simulink model "simulazione"  (R2021b)
settings: Solver=FixedStepAuto  StartTime=0.0  StopTime=1000  FixedStep=0.001  RelTol=1e-3
values from neighbouring files (symbols this model uses):
  b1 = 0.3    [linearizzazione.m]    (also in progetto.m)
  b2 = 0.1    [linearizzazione.m]    (also in progetto.m)
  DD = 3e-5    (= 3e-05)    [progetto.m]
  k = 1.5    [linearizzazione.m]    (also in progetto.m)
  kG = 6.67e-11    [linearizzazione.m]    (also in progetto.m)
  m = 1    [linearizzazione.m]    (also in progetto.m)
  M = 5.98e24    (= 5.98e+24)    [linearizzazione.m]    (also in progetto.m)
  u_e = 364.63    [linearizzazione.m]    (also in progetto.m)
  WW = 8e-5    (= 8e-05)    [progetto.m]
  x1_e = 3e7    (= 30000000)    [linearizzazione.m]    (also in progetto.m)
  x2_e = 0    [linearizzazione.m]    (also in progetto.m)
  x3_e = 0.000121543    [linearizzazione.m]    (also in progetto.m)
undefined symbols (not defined in the file or in its folder): NN
settings Model: Creator=lollo  LastModifiedBy=lollo

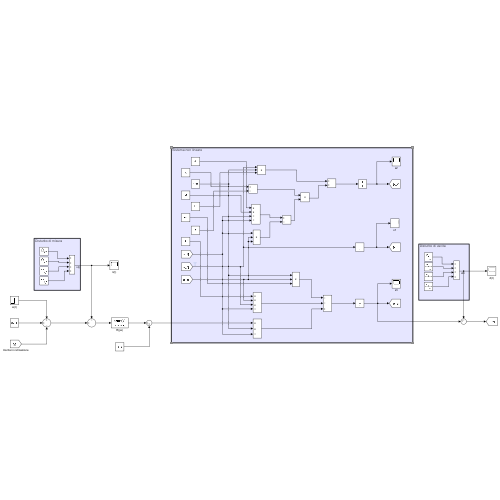
[thumbnail: Simulink's stored preview of the top-level diagram]
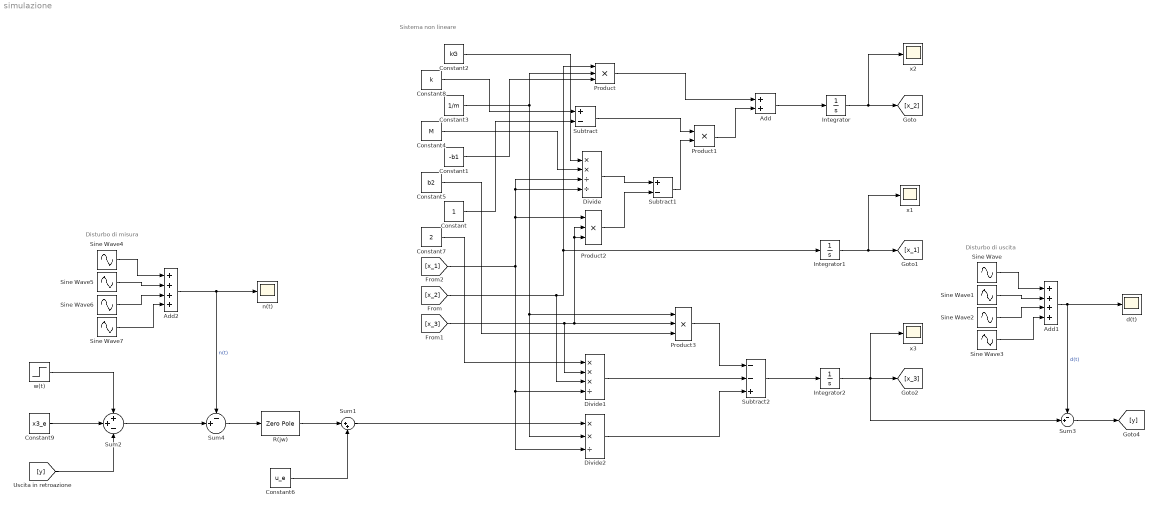
== system simulazione ==
  note: Sistema non lineare
  note: Disturbo di uscita
  note: Disturbo di misura
  Add : Sum
  Add1 : Sum  Inputs=++++
  Add2 : Sum  Inputs=++++
  Constant : Constant
  Constant1 : Constant  Value=-b1
  Constant2 : Constant  Value=kG
  Constant3 : Constant  Value=1/m
  Constant4 : Constant  Value=M
  Constant5 : Constant  Value=b2
  Constant6 : Constant  Value=u_e
  Constant7 : Constant  Value=2
  Constant8 : Constant  Value=k
  Constant9 : Constant  Value=x3_e
  Divide : Product  Inputs=**//
  Divide1 : Product  Inputs=***/
  Divide2 : Product  Inputs=**/
  Integrator : Integrator  InitialCondition=x2_e
  Integrator1 : Integrator  InitialCondition=x1_e
  Integrator2 : Integrator  InitialCondition=x3_e
  Product : Product  Inputs=3
  Product1 : Product
  Product2 : Product  Inputs=3
  Product3 : Product  Inputs=3
  R(jw) : ZeroPole  Zeros=[-0.3309]  Poles=[0 -830.2822]  Gain=2.5088e12
  Sine Wave : Sin  Amplitude=DD  Frequency=0.02*1  SampleTime=0
  Sine Wave1 : Sin  Amplitude=DD  Frequency=0.02*2  SampleTime=0
  Sine Wave2 : Sin  Amplitude=DD  Frequency=0.02*3  SampleTime=0
  Sine Wave3 : Sin  Amplitude=DD  Frequency=0.02*4  SampleTime=0
  Sine Wave4 : Sin  Amplitude=NN  Frequency=5e4*1  SampleTime=0
  Sine Wave5 : Sin  Amplitude=NN  Frequency=5e4*2  SampleTime=0
  Sine Wave6 : Sin  Amplitude=NN  Frequency=5e4*3  SampleTime=0
  Sine Wave7 : Sin  Amplitude=NN  Frequency=5e4*4  SampleTime=0
  Subtract : Sum  Inputs=+-
  Subtract1 : Sum  Inputs=+-
  Subtract2 : Sum  Inputs=--+
  Sum1 : Sum  Inputs=|++
  Sum2 : Sum  Inputs=++-
  Sum3 : Sum  Inputs=-+|
  Sum4 : Sum  Inputs=-+|
  d(t) : Scope
  n(t) : Scope
  w(t) : Step  Time=0  After=WW  SampleTime=0
  x1 : Scope
  x2 : Scope
  x3 : Scope
  wires:
  Constant1/1 -> Product/3
  Constant3/1 -> Product3/1, Divide2/2, Product/2
  Product/1 -> Add/1
  Constant8/1 -> Subtract/1
  Constant/1 -> Subtract/2
  Subtract/1 -> Product1/1
  Subtract1/1 -> Product1/2
  Constant2/1 -> Divide/1
  Divide/1 -> Subtract1/1
  Integrator/1 -> x2/1, [x_2]
  [x_2] -> Divide1/3, Product/1, Integrator1/1
  Integrator1/1 -> [x_1], x1/1
  Constant4/1 -> Divide/2
  [x_1] -> Divide2/3, Divide1/4, Product2/1, Divide/4, Divide/3
  Product2/1 -> Subtract1/2
  [x_3] -> Divide1/2, Product3/2, Product2/3, Product2/2
  Product1/1 -> Add/2
  Add/1 -> Integrator/1
  Constant7/1 -> Divide1/1
  Divide1/1 -> Subtract2/2
  Constant5/1 -> Product3/3
  Product3/1 -> Subtract2/1
  Divide2/1 -> Subtract2/3
  Subtract2/1 -> Integrator2/1
  Integrator2/1 -> Sum3/2, [x_3], x3/1
  R(jw)/1 -> Sum1/1
  Constant6/1 -> Sum1/2
  Sum1/1 -> Divide2/1
  Constant9/1 -> Sum2/2
  [y] -> Sum2/3
  Sine Wave/1 -> Add1/1
  Sine Wave1/1 -> Add1/2
  Sine Wave2/1 -> Add1/3
  Sine Wave3/1 -> Add1/4
  Add1/1 -> Sum3/1, d(t)/1  "d(t)"
  Sum3/1 -> [y]
  Sine Wave5/1 -> Add2/2
  Sine Wave6/1 -> Add2/3
  Sine Wave4/1 -> Add2/1
  Sine Wave7/1 -> Add2/4
  Add2/1 -> n(t)/1, Sum4/1  "n(t)"
  Sum2/1 -> Sum4/2
  Sum4/1 -> R(jw)/1
  w(t)/1 -> Sum2/1
